simulink model "SINS_model_3ch_h"  (R2020b)
settings: Solver=FixedStepDiscrete  StartTime=0.0  StopTime=9.99  RelTol=1e-3
settings Model: Creator=Kolganov  LastModifiedBy=leonk
settings DataIOCC: ReturnWorkspaceOutputs=off
settings OptimizationCC: DefaultParameterBehavior=Inlined  InlineInvariantSignals=on  PassReuseOutputArgsAs=Individual arguments  ZeroExternalMemoryAtStartup=off  ZeroInternalMemoryAtStartup=off  NoFixptDivByZeroProtection=on  EfficientFloat2IntCast=on  LifeSpan=1  OptimizeBlockOrder=speed  OptimizationPriority=Speed  EfficientTunableParamExpr=on
settings DebuggingCC: ParameterTunabilityLossMsg=error  UnderSpecifiedDimensionMsg=warning  ArithmeticOperatorsInVariantConditions=warning
settings HardwareCC: ProdBitPerPointer=32  ProdBitPerSizeT=32  ProdBitPerPtrDiffT=32  ProdLargestAtomicInteger=Long  ProdLargestAtomicFloat=Double  ProdWordSize=32  ProdLongLongMode=on  ProdHWDeviceType=NXP->Cortex-M4
settings SFSimCC: SimUseLocalCustomCode=off  MATLABDynamicMemAlloc=off  CustomCodeUndefinedFunction=UseInterfaceOnly
settings RTWCC: Description=Embedded Coder  SystemTargetFile=ert.tlc  GenCodeOnly=on  TemplateMakefile=ert_default_tmf  GenerateReport=on  RTWUseLocalCustomCode=off  BuildConfiguration=Faster Runs  IncludeHyperlinkInReport=on  LaunchReport=on  GenerateTraceInfo=on  GenerateTraceReport=on  GenerateTraceReportSl=on  GenerateTraceReportSf=on  GenerateTraceReportEml=on  GenerateCodeMetricsReport=on
settings CodeAppCC: ForceParamTrailComments=on  IgnoreCustomStorageClasses=off  OperatorAnnotations=on  SimulinkDataObjDesc=on  SFDataObjDesc=on  InsertBlockDesc=on
settings ERTTargetCC: TargetLangStandard=C99 (ISO)  GenerateFullHeader=off  GenerateSampleERTMain=on  IncludeMdlTerminateFcn=off  CombineSignalStateStructs=on  ERTCustomFileBanners=off  SupportAbsoluteTime=off  SupportNonFinite=off  SupportComplex=off  SupportNonInlinedSFcns=on  ParenthesesLevel=Minimum  InlinedParameterPlacement=NonHierarchical  ERTCustomFileTemplate=example_file_process.tlc  ERTFilePackagingFormat=CompactWithDataFile  IndentSize=4

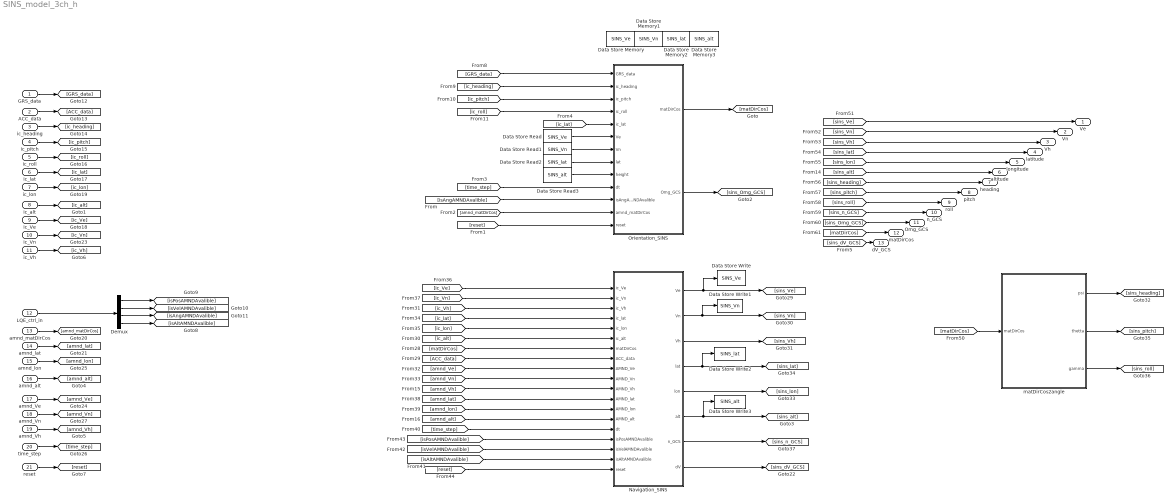
== system SINS_model_3ch_h ==
  GRS_data : Inport  PortDimensions=[3,1]
  ACC_data : Inport  Port=2  PortDimensions=[3,1]
  ic_heading : Inport  Port=3  PortDimensions=1
  ic_pitch : Inport  Port=4  PortDimensions=1
  ic_roll : Inport  Port=5  PortDimensions=1
  ic_lat : Inport  Port=6  PortDimensions=1
  ic_lon : Inport  Port=7  PortDimensions=1
  ic_alt : Inport  Port=8  PortDimensions=1
  ic_Ve : Inport  Port=9  PortDimensions=1
  ic_Vn : Inport  Port=10  PortDimensions=1
  ic_Vh : Inport  Port=11  PortDimensions=1
  LQE_ctrl_in : Inport  Port=12  PortDimensions=[4,1]
  amnd_matDirCos : Inport  Port=13  PortDimensions=[3,3]
  amnd_lat : Inport  Port=14  PortDimensions=1
  amnd_lon : Inport  Port=15
  amnd_alt : Inport  Port=16
  amnd_Ve : Inport  Port=17  PortDimensions=1
  amnd_Vn : Inport  Port=18  PortDimensions=1
  amnd_Vh : Inport  Port=19  PortDimensions=1
  time_step : Inport  Port=20  PortDimensions=1
  reset : Inport  Port=21  PortDimensions=1
  Data Store Memory : DataStoreMemory  DataStoreName=SINS_Ve  ShowAdditionalParam=off
  Data Store Memory1 : DataStoreMemory  DataStoreName=SINS_Vn  ShowAdditionalParam=off
  Data Store Memory2 : DataStoreMemory  DataStoreName=SINS_lat  ShowAdditionalParam=off
  Data Store Memory3 : DataStoreMemory  DataStoreName=SINS_alt  ShowAdditionalParam=off
  Data Store Read : DataStoreRead  DataStoreName=SINS_Ve
  Data Store Read1 : DataStoreRead  DataStoreName=SINS_Vn
  Data Store Read2 : DataStoreRead  DataStoreName=SINS_lat
  Data Store Read3 : DataStoreRead  DataStoreName=SINS_alt
  Data Store Write : DataStoreWrite  DataStoreName=SINS_Ve
  Data Store Write1 : DataStoreWrite  DataStoreName=SINS_Vn
  Data Store Write2 : DataStoreWrite  DataStoreName=SINS_lat
  Data Store Write3 : DataStoreWrite  DataStoreName=SINS_alt
  Demux : Demux
  Navigation_SINS : MATLAB Function  TreatAsAtomicUnit=on
  Orientation_SINS : MATLAB Function  TreatAsAtomicUnit=on
  matDirCos2angle : MATLAB Function  TreatAsAtomicUnit=on
  Ve : Outport  PortDimensions=1  VectorParamsAs1DForOutWhenUnconnected=off
  Vn : Outport  Port=2  PortDimensions=1  VectorParamsAs1DForOutWhenUnconnected=off
  Vh : Outport  Port=3  PortDimensions=1  VectorParamsAs1DForOutWhenUnconnected=off
  latitude : Outport  Port=4  PortDimensions=1  VectorParamsAs1DForOutWhenUnconnected=off
  longitude : Outport  Port=5  PortDimensions=1  VectorParamsAs1DForOutWhenUnconnected=off
  altitude : Outport  Port=6  PortDimensions=1  VectorParamsAs1DForOutWhenUnconnected=off
  heading : Outport  Port=7  VectorParamsAs1DForOutWhenUnconnected=off
  pitch : Outport  Port=8  VectorParamsAs1DForOutWhenUnconnected=off
  roll : Outport  Port=9  VectorParamsAs1DForOutWhenUnconnected=off
  n_GCS : Outport  Port=10  PortDimensions=[3,1]  VectorParamsAs1DForOutWhenUnconnected=off
  Omg_GCS : Outport  Port=11  PortDimensions=[3,1]  VectorParamsAs1DForOutWhenUnconnected=off
  matDirCos : Outport  Port=12  PortDimensions=[3,3]  VectorParamsAs1DForOutWhenUnconnected=off
  dV_GCS : Outport  Port=13  PortDimensions=[3,1]  VectorParamsAs1DForOutWhenUnconnected=off
  wires:
  GRS_data/1 -> [GRS_data]
  ACC_data/1 -> [ACC_data]
  ic_heading/1 -> [ic_heading]
  ic_roll/1 -> [ic_roll]
  ic_pitch/1 -> [ic_pitch]
  ic_lat/1 -> [ic_lat]
  ic_lon/1 -> [ic_lon]
  ic_Ve/1 -> [ic_Ve]
  amnd_lat/1 -> [amnd_lat]
  amnd_matDirCos/1 -> [amnd_matDirCos]
  LQE_ctrl_in/1 -> Demux/1
  ic_Vn/1 -> [ic_Vn]
  amnd_Ve/1 -> [amnd_Ve]
  amnd_lon/1 -> [amnd_lon]
  amnd_Vn/1 -> [amnd_Vn]
  time_step/1 -> [time_step]
  ic_alt/1 -> [ic_alt]
  ic_Vh/1 -> [ic_Vh]
  Demux/1 -> [isPosAMNDAvalible]
  Demux/2 -> [isVelAMNDAvalible]
  Demux/3 -> [isAngAMNDAvalible]
  [matDirCos] -> Navigation_SINS/7(matDirCos)
  [ACC_data] -> Navigation_SINS/8(ACC_data)
  [amnd_Ve] -> Navigation_SINS/9(AMND_Ve)
  [amnd_Vn] -> Navigation_SINS/10(AMND_Vn)
  [ic_lat] -> Navigation_SINS/4(ic_lat)
  [ic_lon] -> Navigation_SINS/5(ic_lon)
  [ic_Ve] -> Navigation_SINS/1(ic_Ve)
  [ic_Vn] -> Navigation_SINS/2(ic_Vn)
  [amnd_lat] -> Navigation_SINS/12(AMND_lat)
  [amnd_lon] -> Navigation_SINS/13(AMND_lon)
  [time_step] -> Navigation_SINS/15(dt)
  [isVelAMNDAvalible] -> Navigation_SINS/17(isVelAMNDAvalible)
  [isPosAMNDAvalible] -> Navigation_SINS/16(isPosAMNDAvalible)
  [reset] -> Navigation_SINS/19(reset)
  Navigation_SINS/3(Vh) -> [sins_Vh]
  Navigation_SINS/5(lon) -> [sins_lon]
  Navigation_SINS/4(lat) -> [sins_lat], Data Store Write2/1
  [matDirCos] -> matDirCos2angle/1(matDirCos)
  matDirCos2angle/3(gamma) -> [sins_roll]
  matDirCos2angle/2(thetta) -> [sins_pitch]
  [sins_Ve] -> Ve/1
  [sins_Vn] -> Vn/1
  [sins_Vh] -> Vh/1
  [sins_lat] -> latitude/1
  [sins_lon] -> longitude/1
  [sins_heading] -> heading/1
  [sins_roll] -> roll/1
  [sins_pitch] -> pitch/1
  [sins_n_GCS] -> n_GCS/1
  [sins_Omg_GCS] -> Omg_GCS/1
  [matDirCos] -> matDirCos/1
  Navigation_SINS/7(n_GCS) -> [sins_n_GCS]
  [isAngAMNDAvalible] -> Orientation_SINS/11(isAngAMNDAvalible)
  [reset] -> Orientation_SINS/13(reset)
  [amnd_matDirCos] -> Orientation_SINS/12(amnd_matDirCos)
  [time_step] -> Orientation_SINS/10(dt)
  [GRS_data] -> Orientation_SINS/1(GRS_data)
  Orientation_SINS/2(Omg_GCS) -> [sins_Omg_GCS]
  [ic_pitch] -> Orientation_SINS/3(ic_pitch)
  [ic_roll] -> Orientation_SINS/4(ic_roll)
  Orientation_SINS/1(matDirCos) -> [matDirCos]
  Navigation_SINS/1(Ve) -> Data Store Write/1, [sins_Ve]
  Navigation_SINS/2(Vn) -> [sins_Vn], Data Store Write1/1
  [ic_heading] -> Orientation_SINS/2(ic_heading)
  matDirCos2angle/1(psi) -> [sins_heading]
  Navigation_SINS/6(alt) -> [sins_alt], Data Store Write3/1
  [sins_alt] -> altitude/1
  [ic_alt] -> Navigation_SINS/6(ic_alt)
  [ic_Vh] -> Navigation_SINS/3(ic_Vh)
  amnd_alt/1 -> [amnd_alt]
  amnd_Vh/1 -> [amnd_Vh]
  [amnd_Vh] -> Navigation_SINS/11(AMND_Vh)
  [amnd_alt] -> Navigation_SINS/14(AMND_alt)
  Demux/4 -> [isAltAMNDAvalible]
  [isAltAMNDAvalible] -> Navigation_SINS/18(isAltAMNDAvalible)
  reset/1 -> [reset]
  Data Store Read2/1 -> Orientation_SINS/8(lat)
  Data Store Read3/1 -> Orientation_SINS/9(height)
  Data Store Read1/1 -> Orientation_SINS/7(Vn)
  Data Store Read/1 -> Orientation_SINS/6(Ve)
  [ic_lat] -> Orientation_SINS/5(ic_lat)
  Navigation_SINS/8(dV) -> [sins_dV_GCS]
  [sins_dV_GCS] -> dV_GCS/1

== matlab function SINS_model_3ch_h/matDirCos2angle ==
  data: matDirCos input; psi output; thetta output; gamma output
function [psi, thetta, gamma] = matDirCos2angle(matDirCos)

    psi = 0;%курс
    thetta = 0;%тангаж
    gamma = 0;%крен
    
    
%--------------------------------------------------------------------------
    %heading     
    
    if (matDirCos(2,1) > (sqrt(2)/2))
        psi = atan2(matDirCos(1,1), matDirCos(2,1));
    else 
        psi = pi/2 - atan2(matDirCos(2,1), matDirCos(1,1));
    end
  
    if (psi < 0)
        psi = psi + 2*pi;
    end

    if (psi > 2*pi)
        psi = psi - 2*pi;
    end
    
%--------------------------------------------------------------------------
    %pitch
    
    thetta = asin(matDirCos(3,1));
   
    if (thetta > pi/2)
        thetta = pi - thetta;
    end
    if (thetta < -pi/2)
        thetta = - pi - thetta;
    end
    
%--------------------------------------------------------------------------
    %roll
    
    if (matDirCos(3,2) > (sqrt(2)/2))
        gamma = atan2(-matDirCos(3,3), matDirCos(3,2));
    else 
        gamma = pi/2 - atan2(matDirCos(3,2), -matDirCos(3,3));
    end
    if (gamma > pi)
        gamma = -2*pi + gamma;
    end

    if (gamma < -pi)
        gamma = 2*pi + gamma; 
    end

== matlab function SINS_model_3ch_h/Orientation_SINS ==
  data: GRS_data input; ic_heading input; ic_pitch input; ic_roll input; ic_lat input; Ve input; matDirCos output; Vn input; Omg_GCS output; lat input; height input; dt input; isAngAMNDAvalible input; amnd_matDirCos input; reset input
function [matDirCos, Omg_GCS]= fcn(GRS_data, ic_heading, ic_pitch,...
        ic_roll, ic_lat,Ve, Vn,lat, height,dt,...
        isAngAMNDAvalible,amnd_matDirCos,reset)

    persistent matDirCos_mem
    if isempty(matDirCos_mem)||(reset == 1)
        matDirCos_mem = zeros(3,3) + get_ic_matDirCos(ic_heading,ic_pitch...
                                                                 ,ic_roll);
        lat = ic_lat;
    end
    
%     if isAngAMNDAvalible == 1
% %         matDirCos_mem  =  amnd_matDirCos*matDirCos_mem; 
%         matDirCos_mem = matDirCos_mem - amnd_matDirCos*matDirCos_mem;
% %         matDirCos_mem = get_ic_matDirCos(amnd_matDirCos(1,1),amnd_matDirCos(2,1), amnd_matDirCos(3,1));
%     end   
%--------------------------------------------------------------------------      
    matDirCos = zeros(3,3);
    Omg_GCS   = zeros(3,1);
%--------------------------------------------------------------------------    
    a = 6378136;
    e2 = 0.0066943662;
    U = deg2rad (360 / (23 * 3600 + 56 * 60  + 4.09));%(15/3600)*pi/180;
    Un = U*cos(lat);
    Uh = U*sin(lat);
%--------------------------------------------------------------------------
    Omega_x = GRS_data(1);%0;
    Omega_y = GRS_data(2);%0;  
    Omega_z = GRS_data(3);%U; 
%--------------------------------------------------------------------------
    ro_1 = a*(1-e2)/(1-e2*sin(lat)^2)^(3/2) + height;% (rm + h)
    ro_2 = a*(1-e2*sin(lat)^2)^(-1/2) + height;% (rn + h)
%--------------------------------------------------------------------------    
    omega_e = -Vn/ro_1;
    omega_n =  Ve/ro_2;
    omega_h = (Ve/ro_2)*tan(lat);

    Omega_gor =  [0            , -(omega_h + Uh),  (omega_n + Un);
                 (omega_h + Uh),  0             , -(omega_e)     ;
                -(omega_n + Un),  (omega_e)     ,  0            ];
            
    Omg_GCS = [omega_e;omega_n + Un;omega_h + Uh];
    
    Omega_gyro =  [0      , -Omega_z,  Omega_y;
                   Omega_z,  0      , -Omega_x;
                  -Omega_y,  Omega_x,  0     ];
         
    d_matDirCos = matDirCos_mem*Omega_gyro - Omega_gor*matDirCos_mem;
       
    matDirCos_mem = matDirCos_mem + d_matDirCos*dt;
%-------------------------------------------------------------------------- 
 
%--------------------------------------------------------------------------       
            
    [U,~,V] = svd(matDirCos_mem);
    matDirCos_mem = U * V';
%--------------------------------------------------------------------------   
    matDirCos = matDirCos_mem;
end
%==========================================================================
function ic_matDirCos = get_ic_matDirCos(psi,theta,gamma)
%yaw
%ic_matDirCos = [-sin(psi)*cos(theta),  sin(psi)*sin(theta)*cos(gamma)+cos(psi)*sin(gamma), -sin(psi)*sin(theta)*sin(gamma) + cos(psi)*cos(gamma);
%                 cos(psi)*cos(theta), -cos(psi)*sin(theta)*cos(gamma)+sin(psi)*sin(gamma),  cos(psi)*sin(theta)*sin(gamma) - sin(psi)*cos(gamma);
%                 sin(theta)         ,  cos(theta)*cos(gamma)                             , -cos(theta)*sin(gamma)                               ];

%heading
ic_matDirCos = [sin(psi)*cos(theta), -sin(psi)*sin(theta)*cos(gamma)+cos(psi)*sin(gamma),  sin(psi)*sin(theta)*sin(gamma) + cos(psi)*cos(gamma);
                cos(psi)*cos(theta), -cos(psi)*sin(theta)*cos(gamma)-sin(psi)*sin(gamma),  cos(psi)*sin(theta)*sin(gamma) - sin(psi)*cos(gamma);
                sin(theta)         ,  cos(theta)*cos(gamma)                             , -cos(theta)*sin(gamma)                               ];
end

== matlab function SINS_model_3ch_h/Navigation_SINS ==
  data: ic_Ve input; Ve output; Vn output; ic_Vn input; ic_Vh input; ic_lat input; ic_lon input; ic_alt input; matDirCos input; ACC_data input; AMND_Ve input; AMND_Vn input; AMND_Vh input; AMND_lat input; AMND_lon input; AMND_alt input; dt input; isPosAMNDAvalible input; isVelAMNDAvalible input; isAltAMNDAvalible input; reset input; Vh output; lat output; lon output; alt output; n_GCS output; dV output
function [Ve, Vn, Vh, lat, lon, alt, n_GCS, dV] = calc_navigation...
                (ic_Ve, ic_Vn, ic_Vh, ic_lat, ic_lon,ic_alt, ...
                 matDirCos, ACC_data,...
                 AMND_Ve, AMND_Vn,AMND_Vh, AMND_lat, AMND_lon,AMND_alt,...
                 dt,...
                 isPosAMNDAvalible, isVelAMNDAvalible, isAltAMNDAvalible,...
                 reset)
%--------------------------------------------------------------------------

Vh = ic_Vh;
    persistent Ve_mem Vn_mem Vh_mem lat_mem lon_mem alt_mem  
    %Omega_E Omega_N Omega_H
    if isempty(Ve_mem)||(reset == 1)
        
        Ve_mem  = ic_Ve;
        Vn_mem  = ic_Vn;
        Vh_mem  = ic_Vh;
        lat_mem = ic_lat;
        lon_mem = ic_lon;        
        alt_mem = ic_alt;
     
    end
%--------------------------------------------------------------------------    
    beta  = double(0.0053171);
    beta1 = double(71*10^-7);
    q     = double(0.00346775);
    ge    = double(9.78049);
    a     = double(6378136);                                                           %PZ-90
    e2    = double(0.0066943662); 
%--------------------------------------------------------------------------
     if isPosAMNDAvalible == 1
        lat_mem = lat_mem - AMND_lat;
        lon_mem = lon_mem - AMND_lon;      
     end
    if isVelAMNDAvalible == 1
        Ve_mem = Ve_mem - AMND_Ve;
        Vn_mem = Vn_mem - AMND_Vn;
     end
     if isAltAMNDAvalible == 1
        alt_mem = alt_mem - AMND_alt;
        Vh_mem = Vh_mem   - AMND_Vh;  
     end

    U = deg2rad (360 / (23 * 3600 + 56 * 60  + 4.09));
    Un = U*cos(lat_mem);
    Uh = U*sin(lat_mem);
%--------------------------------------------------------------------------   
    n_GCS = zeros(3,1);
    n_GCS = matDirCos*ACC_data;   
    n_e = n_GCS(1); n_n = n_GCS(2); n_h = n_GCS(3);                        
%Erath radius

    ro_1 = a*(1-e2)/(1-e2*sin(lat_mem)^2)^(3/2) + alt_mem;% (rm + h)
    ro_2 = a*(1-e2*sin(lat_mem)^2)^(-1/2) + alt_mem;% (rn + h)
    
%velocity in [rad/s]
    Omega_E = -Vn_mem/ro_1; 
    Omega_N =  Ve_mem/ro_2;
    Omega_H = (Ve_mem/ro_2)*tan(lat_mem);   
    
    r_lon = cos(lat_mem)*ro_2;
    r_lat = ro_1;

%centripetal acceleration from Chekhov's book    
    centr_acc =[- sin(lat_mem)*r_lon*(U)^2;...
                  cos(lat_mem)*r_lon*(U)^2;...
                  0];
    
    g0 = ge*(1 + beta*sin(lat_mem)^2 + beta1*sin(2*lat_mem)^2);
    gn = g0*sin(2*lat_mem)*(alt_mem/a)*((e2)/a - 2*q);
    gh = g0 + (alt_mem/a)*((3*alt_mem/a) - 2*q*ge*cos(lat_mem)^2 + ...
                 (e2)*(3*sin(lat_mem)^2 - 1) - q*(1+6*sin(lat_mem)^2));
               
    acc_e = 0  - centr_acc(3);
    acc_n = gn - centr_acc(1);
    acc_h = gh - centr_acc(2);
  
%--------------------------------------------------------------------------   
    matr_Omega = [ 0,        Omega_H, -Omega_N;...
                  -Omega_H,  0,        Omega_E;...
                   Omega_N, -Omega_E,  0];
    matr_U     = [ 0,  Uh, -Un;...
                  -Uh, 0,   0;...
                   Un, 0,   0];
               
    dV     = (matr_Omega + 2*matr_U)*[Ve_mem;Vn_mem;Vh_mem] + ...
             [n_e; n_n; n_h] - [acc_e;acc_n;acc_h];
    
    
    Ve_mem = Ve_mem + dV(1)*dt;
    Vn_mem = Vn_mem + dV(2)*dt;
    Vh_mem = Vh_mem + dV(3)*dt;
    
    Omega_E = -Vn_mem/ro_1; 
    Omega_N =  Ve_mem/ro_2;
    Omega_H = (Ve_mem/ro_2)*tan(lat_mem);   
    
    dLat    = -Omega_E;
    dLon    =  Omega_N/cos(lat_mem);
    
    lat_mem = lat_mem + dLat*dt   + ((dV(2)/ro_1)*dt^2)/2 ;
    lon_mem = lon_mem + dLon*dt   + ((dV(1)/ro_2)*dt^2)/2;
    alt_mem = alt_mem + Vh_mem*dt + ((dV(3)*dt^2))/2;
    
    Ve  = Ve_mem ; Vn  = Vn_mem ; Vh = Vh_mem;         
    lat = lat_mem; lon = lon_mem; alt = alt_mem;


    
end
